simulink model "Modelisation_3_MG_MC_MA_Comparaison_avec_SimMechanics"  (R2016a)
settings: Solver=ode45  StartTime=0.0  StopTime=2.5  RelTol=1e-3
values from neighbouring files (symbols this model uses):
  s = tf('s')    [A_3_LoopShaping.m]    (also in A_4_Hinfini.m = zpk('s'))
  X = [0;0;0;0;0;0;0;0]    [A_1_Data.m]
  Y = [0;0;0;0;0;0;0;0]    [A_1_Data.m]
undefined symbols (not defined in the file or in its folder): sfun3d, Z
libraries: sm_lib x280, nesl_utility x16
(part 7 of 7)

== system Modelisation_3_MG_MC_MA_Comparaison_avec_SimMechanics/SM/Subsystem5/BarreParalleles_3_RIGID/Pi_ce4_Extremetees_1_RIGID ==
  ReferenceFrame : sm_lib/Frames and Transforms/Reference Frame
  Solid : sm_lib/Body Elements/Solid  InertiaType=Custom  Mass=0.0043409919402835973  MassUnits=kg  CenterOfMass=[-6.6394731008193298e-06 -1.3723999560385904 4.9969803448403587]  CenterOfMassUnits=mm  MomentsOfInertia=[0.22208105944838133 0.24049053699814107 0.066049415613599144]  MomentsOfInertiaUnits=kg*mm^2  ProductsOfInertia=[-0.022728057317176146 1.1398156711537084e-07 7.9844492116540505e-07]  ProductsOfInertiaUnits=kg*mm^2  DensityBased=on  Density=1000  DensityUnits=kg/(m^3)  DoExposeReferenceFrame=on  SerializedFrames=<Frames/>  GraphicType=FromGeometry  MarkerShape=Sphere  MarkerSize=10  MarkerSizeUnits=m  GraphicVisPropType=SimpleVisualProperties  GraphicDiffuseColor=[0.59999999999999998 0.59999999999999998 0.59999999999999998]  GraphicSpecularColor=[0.5 0.5 0.5 1.0]  GraphicAmbientColor=[0.15 0.15 0.15 1.0]  GraphicEmissiveColor=[0.0 0.0 0.0 1.0]  GraphicShininess=75  GraphicOpacity=1  GeometryShape=FromFile  RectangleSize=[1 1]  RectangleSizeUnits=m  BrickDimensions=[1 1 1]  BrickDimensionUnits=m  CylinderRadius=1  CylinderRadiusUnits=m  CylinderLength=1  CylinderLengthUnits=m  SphereRadius=1  SphereRadiusUnits=m  EllipsoidRadii=[1 1 1]  EllipsoidRadiiUnits=m  ExtrusionCrossSection=[1 1; -1 1; -1 -1; 1 -1]  ExtrusionCrossSectionUnits=m  ExtrusionLength=1  ExtrusionLengthUnits=m  PolygonNumSides=3  PolygonOuterRadius=1  PolygonOuterRadiusUnits=m  ExtGeomFileType=STL  ExtGeomFileName=Pièce4_Extremetees_Défaut_sldprt.STL  ExtGeomFileUnits=mm  RevolutionCrossSection=[1 1; 1 -1; 2 -1; 2 1]  RevolutionCrossSectionUnits=m  RevolutionExtent=Full  RevolutionAngle=180  RevolutionAngleUnits=deg
  F : PMIOPort  Port=1  Side=Left
  connections:
  F/RConn1 -- ReferenceFrame/RConn1 -- Solid/RConn1

== system Modelisation_3_MG_MC_MA_Comparaison_avec_SimMechanics/SM/Subsystem5/BarreParalleles_3_RIGID/Pi_ce4_Extremetees_2_RIGID ==
  ReferenceFrame : sm_lib/Frames and Transforms/Reference Frame
  Solid : sm_lib/Body Elements/Solid  InertiaType=Custom  Mass=0.0043409919402835973  MassUnits=kg  CenterOfMass=[-6.6394731008193298e-06 -1.3723999560385904 4.9969803448403587]  CenterOfMassUnits=mm  MomentsOfInertia=[0.22208105944838133 0.24049053699814107 0.066049415613599144]  MomentsOfInertiaUnits=kg*mm^2  ProductsOfInertia=[-0.022728057317176146 1.1398156711537084e-07 7.9844492116540505e-07]  ProductsOfInertiaUnits=kg*mm^2  DensityBased=on  Density=1000  DensityUnits=kg/(m^3)  DoExposeReferenceFrame=on  SerializedFrames=<Frames/>  GraphicType=FromGeometry  MarkerShape=Sphere  MarkerSize=10  MarkerSizeUnits=m  GraphicVisPropType=SimpleVisualProperties  GraphicDiffuseColor=[0.59999999999999998 0.59999999999999998 0.59999999999999998]  GraphicSpecularColor=[0.5 0.5 0.5 1.0]  GraphicAmbientColor=[0.15 0.15 0.15 1.0]  GraphicEmissiveColor=[0.0 0.0 0.0 1.0]  GraphicShininess=75  GraphicOpacity=1  GeometryShape=FromFile  RectangleSize=[1 1]  RectangleSizeUnits=m  BrickDimensions=[1 1 1]  BrickDimensionUnits=m  CylinderRadius=1  CylinderRadiusUnits=m  CylinderLength=1  CylinderLengthUnits=m  SphereRadius=1  SphereRadiusUnits=m  EllipsoidRadii=[1 1 1]  EllipsoidRadiiUnits=m  ExtrusionCrossSection=[1 1; -1 1; -1 -1; 1 -1]  ExtrusionCrossSectionUnits=m  ExtrusionLength=1  ExtrusionLengthUnits=m  PolygonNumSides=3  PolygonOuterRadius=1  PolygonOuterRadiusUnits=m  ExtGeomFileType=STL  ExtGeomFileName=Pièce4_Extremetees_Défaut_sldprt.STL  ExtGeomFileUnits=mm  RevolutionCrossSection=[1 1; 1 -1; 2 -1; 2 1]  RevolutionCrossSectionUnits=m  RevolutionExtent=Full  RevolutionAngle=180  RevolutionAngleUnits=deg
  F : PMIOPort  Port=1  Side=Left
  connections:
  F/RConn1 -- ReferenceFrame/RConn1 -- Solid/RConn1

== system Modelisation_3_MG_MC_MA_Comparaison_avec_SimMechanics/SM/Subsystem5/BarreParalleles_3_RIGID/Pi_ce4_Tube_1_RIGID ==
  ReferenceFrame : sm_lib/Frames and Transforms/Reference Frame
  Solid : sm_lib/Body Elements/Solid  InertiaType=Custom  Mass=0.0056953775725032503  MassUnits=kg  CenterOfMass=[-4.1460122344799134e-11 2.6332345173922464e-08 157.00037492761294]  CenterOfMassUnits=mm  MomentsOfInertia=[46.656669534748204 46.656784060773653 0.060513437161415488]  MomentsOfInertiaUnits=kg*mm^2  ProductsOfInertia=[4.4271388779002391e-06 -1.0344554341986986e-06 -6.5578304138838094e-07]  ProductsOfInertiaUnits=kg*mm^2  DensityBased=on  Density=1000  DensityUnits=kg/(m^3)  DoExposeReferenceFrame=on  SerializedFrames=<Frames/>  GraphicType=FromGeometry  MarkerShape=Sphere  MarkerSize=10  MarkerSizeUnits=m  GraphicVisPropType=SimpleVisualProperties  GraphicDiffuseColor=[1 1 1]  GraphicSpecularColor=[0.5 0.5 0.5 1.0]  GraphicAmbientColor=[0.15 0.15 0.15 1.0]  GraphicEmissiveColor=[0.0 0.0 0.0 1.0]  GraphicShininess=75  GraphicOpacity=1  GeometryShape=FromFile  RectangleSize=[1 1]  RectangleSizeUnits=m  BrickDimensions=[1 1 1]  BrickDimensionUnits=m  CylinderRadius=1  CylinderRadiusUnits=m  CylinderLength=1  CylinderLengthUnits=m  SphereRadius=1  SphereRadiusUnits=m  EllipsoidRadii=[1 1 1]  EllipsoidRadiiUnits=m  ExtrusionCrossSection=[1 1; -1 1; -1 -1; 1 -1]  ExtrusionCrossSectionUnits=m  ExtrusionLength=1  ExtrusionLengthUnits=m  PolygonNumSides=3  PolygonOuterRadius=1  PolygonOuterRadiusUnits=m  ExtGeomFileType=STL  ExtGeomFileName=Pièce4_Tube_Défaut_sldprt.STL  ExtGeomFileUnits=mm  RevolutionCrossSection=[1 1; 1 -1; 2 -1; 2 1]  RevolutionCrossSectionUnits=m  RevolutionExtent=Full  RevolutionAngle=180  RevolutionAngleUnits=deg
  F : PMIOPort  Port=1  Side=Left
  connections:
  F/RConn1 -- ReferenceFrame/RConn1 -- Solid/RConn1

== system Modelisation_3_MG_MC_MA_Comparaison_avec_SimMechanics/SM/Subsystem5/BarreParalleles_4_RIGID/Pi_ce4_Extremetees_1_RIGID ==
  ReferenceFrame : sm_lib/Frames and Transforms/Reference Frame
  Solid : sm_lib/Body Elements/Solid  InertiaType=Custom  Mass=0.0043409919402835973  MassUnits=kg  CenterOfMass=[-6.6394731008193298e-06 -1.3723999560385904 4.9969803448403587]  CenterOfMassUnits=mm  MomentsOfInertia=[0.22208105944838133 0.24049053699814107 0.066049415613599144]  MomentsOfInertiaUnits=kg*mm^2  ProductsOfInertia=[-0.022728057317176146 1.1398156711537084e-07 7.9844492116540505e-07]  ProductsOfInertiaUnits=kg*mm^2  DensityBased=on  Density=1000  DensityUnits=kg/(m^3)  DoExposeReferenceFrame=on  SerializedFrames=<Frames/>  GraphicType=FromGeometry  MarkerShape=Sphere  MarkerSize=10  MarkerSizeUnits=m  GraphicVisPropType=SimpleVisualProperties  GraphicDiffuseColor=[0.59999999999999998 0.59999999999999998 0.59999999999999998]  GraphicSpecularColor=[0.5 0.5 0.5 1.0]  GraphicAmbientColor=[0.15 0.15 0.15 1.0]  GraphicEmissiveColor=[0.0 0.0 0.0 1.0]  GraphicShininess=75  GraphicOpacity=1  GeometryShape=FromFile  RectangleSize=[1 1]  RectangleSizeUnits=m  BrickDimensions=[1 1 1]  BrickDimensionUnits=m  CylinderRadius=1  CylinderRadiusUnits=m  CylinderLength=1  CylinderLengthUnits=m  SphereRadius=1  SphereRadiusUnits=m  EllipsoidRadii=[1 1 1]  EllipsoidRadiiUnits=m  ExtrusionCrossSection=[1 1; -1 1; -1 -1; 1 -1]  ExtrusionCrossSectionUnits=m  ExtrusionLength=1  ExtrusionLengthUnits=m  PolygonNumSides=3  PolygonOuterRadius=1  PolygonOuterRadiusUnits=m  ExtGeomFileType=STL  ExtGeomFileName=Pièce4_Extremetees_Défaut_sldprt.STL  ExtGeomFileUnits=mm  RevolutionCrossSection=[1 1; 1 -1; 2 -1; 2 1]  RevolutionCrossSectionUnits=m  RevolutionExtent=Full  RevolutionAngle=180  RevolutionAngleUnits=deg
  F : PMIOPort  Port=1  Side=Left
  connections:
  F/RConn1 -- ReferenceFrame/RConn1 -- Solid/RConn1

== system Modelisation_3_MG_MC_MA_Comparaison_avec_SimMechanics/SM/Subsystem5/BarreParalleles_4_RIGID/Pi_ce4_Extremetees_2_RIGID ==
  ReferenceFrame : sm_lib/Frames and Transforms/Reference Frame
  Solid : sm_lib/Body Elements/Solid  InertiaType=Custom  Mass=0.0043409919402835973  MassUnits=kg  CenterOfMass=[-6.6394731008193298e-06 -1.3723999560385904 4.9969803448403587]  CenterOfMassUnits=mm  MomentsOfInertia=[0.22208105944838133 0.24049053699814107 0.066049415613599144]  MomentsOfInertiaUnits=kg*mm^2  ProductsOfInertia=[-0.022728057317176146 1.1398156711537084e-07 7.9844492116540505e-07]  ProductsOfInertiaUnits=kg*mm^2  DensityBased=on  Density=1000  DensityUnits=kg/(m^3)  DoExposeReferenceFrame=on  SerializedFrames=<Frames/>  GraphicType=FromGeometry  MarkerShape=Sphere  MarkerSize=10  MarkerSizeUnits=m  GraphicVisPropType=SimpleVisualProperties  GraphicDiffuseColor=[0.59999999999999998 0.59999999999999998 0.59999999999999998]  GraphicSpecularColor=[0.5 0.5 0.5 1.0]  GraphicAmbientColor=[0.15 0.15 0.15 1.0]  GraphicEmissiveColor=[0.0 0.0 0.0 1.0]  GraphicShininess=75  GraphicOpacity=1  GeometryShape=FromFile  RectangleSize=[1 1]  RectangleSizeUnits=m  BrickDimensions=[1 1 1]  BrickDimensionUnits=m  CylinderRadius=1  CylinderRadiusUnits=m  CylinderLength=1  CylinderLengthUnits=m  SphereRadius=1  SphereRadiusUnits=m  EllipsoidRadii=[1 1 1]  EllipsoidRadiiUnits=m  ExtrusionCrossSection=[1 1; -1 1; -1 -1; 1 -1]  ExtrusionCrossSectionUnits=m  ExtrusionLength=1  ExtrusionLengthUnits=m  PolygonNumSides=3  PolygonOuterRadius=1  PolygonOuterRadiusUnits=m  ExtGeomFileType=STL  ExtGeomFileName=Pièce4_Extremetees_Défaut_sldprt.STL  ExtGeomFileUnits=mm  RevolutionCrossSection=[1 1; 1 -1; 2 -1; 2 1]  RevolutionCrossSectionUnits=m  RevolutionExtent=Full  RevolutionAngle=180  RevolutionAngleUnits=deg
  F : PMIOPort  Port=1  Side=Left
  connections:
  F/RConn1 -- ReferenceFrame/RConn1 -- Solid/RConn1

== system Modelisation_3_MG_MC_MA_Comparaison_avec_SimMechanics/SM/Subsystem5/BarreParalleles_4_RIGID/Pi_ce4_Tube_1_RIGID ==
  ReferenceFrame : sm_lib/Frames and Transforms/Reference Frame
  Solid : sm_lib/Body Elements/Solid  InertiaType=Custom  Mass=0.0056953775725032503  MassUnits=kg  CenterOfMass=[-4.1460122344799134e-11 2.6332345173922464e-08 157.00037492761294]  CenterOfMassUnits=mm  MomentsOfInertia=[46.656669534748204 46.656784060773653 0.060513437161415488]  MomentsOfInertiaUnits=kg*mm^2  ProductsOfInertia=[4.4271388779002391e-06 -1.0344554341986986e-06 -6.5578304138838094e-07]  ProductsOfInertiaUnits=kg*mm^2  DensityBased=on  Density=1000  DensityUnits=kg/(m^3)  DoExposeReferenceFrame=on  SerializedFrames=<Frames/>  GraphicType=FromGeometry  MarkerShape=Sphere  MarkerSize=10  MarkerSizeUnits=m  GraphicVisPropType=SimpleVisualProperties  GraphicDiffuseColor=[1 1 1]  GraphicSpecularColor=[0.5 0.5 0.5 1.0]  GraphicAmbientColor=[0.15 0.15 0.15 1.0]  GraphicEmissiveColor=[0.0 0.0 0.0 1.0]  GraphicShininess=75  GraphicOpacity=1  GeometryShape=FromFile  RectangleSize=[1 1]  RectangleSizeUnits=m  BrickDimensions=[1 1 1]  BrickDimensionUnits=m  CylinderRadius=1  CylinderRadiusUnits=m  CylinderLength=1  CylinderLengthUnits=m  SphereRadius=1  SphereRadiusUnits=m  EllipsoidRadii=[1 1 1]  EllipsoidRadiiUnits=m  ExtrusionCrossSection=[1 1; -1 1; -1 -1; 1 -1]  ExtrusionCrossSectionUnits=m  ExtrusionLength=1  ExtrusionLengthUnits=m  PolygonNumSides=3  PolygonOuterRadius=1  PolygonOuterRadiusUnits=m  ExtGeomFileType=STL  ExtGeomFileName=Pièce4_Tube_Défaut_sldprt.STL  ExtGeomFileUnits=mm  RevolutionCrossSection=[1 1; 1 -1; 2 -1; 2 1]  RevolutionCrossSectionUnits=m  RevolutionExtent=Full  RevolutionAngle=180  RevolutionAngleUnits=deg
  F : PMIOPort  Port=1  Side=Left
  connections:
  F/RConn1 -- ReferenceFrame/RConn1 -- Solid/RConn1

== matlab function Modelisation_3_MG_MC_MA_Comparaison_avec_SimMechanics/SM/MCI ==
  data: alpha input; dalpha input; d2alpha input; alpha_ output; dalpha_ output; d2alpha_ output
    function [alpha_, dalpha_,d2alpha_]= fcn(alpha, dalpha,d2alpha)

   alpha_= -alpha + [0.0651 ; 0.0651 ;0.0651 ] ;  %alpha_= -alpha ;
   dalpha_= -dalpha;
   d2alpha_= -d2alpha ;

== matlab function Modelisation_3_MG_MC_MA_Comparaison_avec_SimMechanics/Modele inverse ==
  data: P input; dP input; d2P input; alpha output; dalpha output; d2alpha output
    function [alpha, dalpha,d2alpha]= fcn(P,dP,d2P)

    l1 = 0.19992; 
    l2 = 0.334; 
    r = 0.126; 
    phi2 = 2*pi/3;
    phi3 = 4*pi/3;

    %% Expression de P dans Ri
    % l'expression P1 dP1 et d2P1 ne se changent pas
    A2=[cos(phi2) sin(phi2) 0
        -sin(phi2) cos(phi2) 0
        0            0      1 ]; 
    A3=[cos(phi3) sin(phi3) 0
        -sin(phi3) cos(phi3) 0
        0            0      1 ];
     P2=A2*P; dP2=A2*dP; d2P2=A2*d2P; 
     P3=A3*P ; dP3=A3*dP ; d2P3=A3*d2P ; 
        
    x1=P(1); y1=P(2) ; z1=P(3) ; 
    x2=P2(1); y2=P2(2) ; z2=P2(3) ;
    x3=P3(1); y3=P3(2) ; z3=P3(3) ;
    % Notation de dP :
    dx1=dP(1); dy1=dP(2) ; dz1=dP(3) ; 
    dx2=dP2(1); dy2=dP2(2) ; dz2=dP2(3) ; 
    dx3=dP3(1); dy3=dP3(2) ; dz3=dP3(3) ; 
    % Notation de d2P :
    d2x1=d2P(1); d2y1=d2P(2) ; d2z1=d2P(3) ;
    d2x2=d2P2(1); d2y2=d2P2(2) ; d2z2=d2P2(3) ;
    d2x3=d2P3(1); d2y3=d2P3(2) ; d2z3=d2P3(3) ;
         

    %% Parametres du Triangle AiCiBi :
    % Triangle 1 :
    AB1=sqrt(z1^2+(x1-r)^2);
    e1=sqrt(l2^2-y1^2); 
    AB2=sqrt(z2^2+(x2-r)^2);
    e2=sqrt(l2^2-y2^2);
    AB3=sqrt(z3^2+(x3-r)^2);
    e3=sqrt(l2^2-y3^2);

    %% calcul de alpha1
    beta1=atan2(-z1,x1-r);
    delta1=acos((AB1^2 + l1^2 - e1^2)/(2*l1*AB1));
    alpha1=beta1-delta1; 


    %% calcul de alpha2
    beta2=atan2(-z2,x2-r);
    delta2=acos((AB2^2 + l1^2 - e2^2)/(2*l1*AB2));
    alpha2=beta2-delta2; 


    %% calcul de alpha3
    beta3=atan2(-z3,x3-r);
    delta3=acos((AB3^2 + l1^2 - e3^2)/(2*l1*AB3));
    alpha3=beta3-delta3; 

% Tranformation au Deg
alpha=[alpha1;alpha2;alpha3]; % first solution


%% =================== Calcule de dalpha_i ====================================

% ---------------------------- Calcul de dAlpha1 ----------------------
% Calcule de dDelta1 :
BH1 = AB1-l1*cos(delta1);
D1=l1*AB1*sin(delta1) ;
dDelta1X = -BH1*(x1-r)/AB1/D1 ; 
dDelta1Y = -y1/D1 ; 
dDelta1Z = -BH1*z1/AB1/D1 ; 
Gdelta1=  [ dDelta1X , dDelta1Y , dDelta1Z] ;
dDelta1 = Gdelta1*dP ;
% Calcule de dBeta1 :
dBeta1Z=-(x1-r)/AB1^2 ; dBeta1X=z1/AB1^2 ;
Gbeta1=[ dBeta1X ,  0 , dBeta1Z] ;
dBeta1 = Gbeta1*dP;
% Calcule de dAlpha1 :
Galpha1=Gbeta1-Gdelta1 ;
dAlpha1 = Galpha1*dP ;

% ---------------------------- Calcul de dAlpha2 ----------------------
% Calcule de dDelta2 :
BH2 = AB2-l1*cos(delta2);
D2=l1*AB2*sin(delta2) ;
dDelta2X = -BH2*(x2-r)/AB2/D2 ; 
dDelta2Y = -y2/D2 ; 
dDelta2Z = -BH2*z2/AB2/D2 ; 
Gdelta2=  [ dDelta2X , dDelta2Y , dDelta2Z] ;
dDelta2 = Gdelta2*dP2 ;
% Calcule de dBeta2 :
dBeta2Z=-(x2-r)/AB2^2 ; dBeta2X=z2/AB2^2 ;
Gbeta2=[ dBeta2X ,  0 , dBeta2Z] ;
dBeta2 = Gbeta2*dP2;
% Calcule de dAlpha2 :
Galpha2=Gbeta2-Gdelta2 ;
dAlpha2 = Galpha2*dP2 ;

% ---------------------------- Calcul de dAlpha3 ----------------------
% Calcule de dDelta2 :
BH3 = AB3-l1*cos(delta3);
D3=l1*AB3*sin(delta3) ;
dDelta3X = -BH3*(x3-r)/AB3/D3 ; 
dDelta3Y = -y3/D3 ; 
dDelta3Z = -BH3*z3/AB3/D3 ; 
Gdelta3=  [ dDelta3X , dDelta3Y , dDelta3Z] ;
dDelta3 = Gdelta3*dP3 ;
% Calcule de dBeta3:
dBeta3Z=-(x3-r)/AB3^2 ; dBeta2X=z3/AB3^2 ;
Gbeta3=[ dBeta2X ,  0 , dBeta3Z] ;
dBeta3 = Gbeta3*dP3;
% Calcule de dAlpha3 :
Galpha3=Gbeta3-Gdelta3 ;
dAlpha3 = Galpha3*dP3 ;

dalpha=[ dAlpha1 ; dAlpha2 ; dAlpha3 ];

%% ===================== Calcule de d2alpha_i =================================
 
% ---------------------------- Calcul de d2Alpha1 ----------------------
% Calcule de d2Gama1 :
CH1=l1*sin(delta1);
AH1=l1*cos(delta1) ;
d2Delta1XX = -BH1*(x1-r)^2/(AB1^3*D1)*( AH1*e1^2/(BH1*CH1^2) + (AB1/(x1-r))^2 - 2 ) ;
d2Delta1YY = - (1+y1^2*AH1*AB1/D1^2 )  /D1;
d2Delta1ZZ  = -BH1*z1^2/(AB1^3*D1)*( AH1*e1^2/(BH1*CH1^2) + (AB1/z1)^2 -2 ) ;
d2Delta1XY = y1*(x1-r)*(CH1^2-AH1*BH1)/D1^3 ;
d2Delta1XZ = -BH1*(x1-r)*z1/(AB1^3*D1)*( AH1*e1^2/(BH1*CH1^2) - 2 ) ;
d2Delta1YZ = y1*z1*(CH1^2-AH1*BH1)/D1^3 ; 
Hdelta1=[ d2Delta1XX,d2Delta1XY,d2Delta1XZ ; d2Delta1XY, d2Delta1YY,d2Delta1YZ ;d2Delta1XZ , d2Delta1YZ,d2Delta1ZZ] ;
d2Delta1=dP'*Hdelta1*dP +  Gdelta1*d2P ; 
%Calcule de dBeta 1:
d2Beta1XX=-2*(x1-r)*z1/AB1^4 ; d2Beta1ZZ=-d2Beta1XX ; d2Beta1XZ = ((x1-r)^2-z1^2)/AB1^4 ;
Hbeta1= [d2Beta1XX , 0, d2Beta1XZ ; 0, 0, 0 ; d2Beta1XZ , 0 , d2Beta1ZZ ] ;
d2Beta1=dP'*Hbeta1*dP + Gbeta1*d2P;
%Calcule de dAlpha1 :
Halpha1= Hbeta1 - Hdelta1; 
d2Alpha1=dP'*Halpha1*dP + Galpha1*d2P;

% ---------------------------- Calcul de d2Alpha2 ----------------------
% Calcule de d2Gama1 :
CH2=l1*sin(delta2);
AH2=l1*cos(delta2) ;
d2Delta2XX = -BH2*(x2-r)^2/(AB2^3*D2)*( AH2*e2^2/(BH2*CH2^2) + (AB2/(x2-r))^2 - 2 ) ;
d2Delta2YY = - (1+y2^2*AH2*AB2/D2^2 )  /D2;
d2Delta2ZZ  = -BH2*z2^2/(AB2^3*D2)*( AH2*e2^2/(BH2*CH2^2) + (AB2/z2)^2 -2 ) ;
d2Delta2XY = y2*(x2-r)*(CH2^2-AH2*BH2)/D2^3 ;
d2Delta2XZ = -BH2*(x2-r)*z2/(AB2^3*D2)*( AH2*e2^2/(BH2*CH2^2) - 2 ) ;
d2Delta2YZ = y2*z2*(CH2^2-AH2*BH2)/D2^3 ; 
Hdelta2=[ d2Delta2XX,d2Delta2XY,d2Delta2XZ ; d2Delta2XY, d2Delta2YY,d2Delta2YZ ;d2Delta2XZ , d2Delta2YZ,d2Delta2ZZ] ;
d2Delta1=dP2'*Hdelta2*dP2 +  Gdelta2*d2P2 ; 
%Calcule de dBeta2:
d2Beta2XX=-2*(x2-r)*z2/AB2^4 ; d2Beta2ZZ=-d2Beta2XX ; d2Beta2XZ = ((x2-r)^2-z2^2)/AB2^4 ;
Hbeta2= [d2Beta2XX , 0, d2Beta2XZ ; 0, 0, 0 ; d2Beta2XZ , 0 , d2Beta2ZZ ] ;
d2Beta2=dP2'*Hbeta2*dP2 + Gbeta2*d2P2;
%Calcule de dAlpha2 :
Halpha2= Hbeta2 - Hdelta2; 
d2Alpha2=dP2'*Halpha2*dP2 + Galpha2*d2P2;

% ---------------------------- Calcul de d2Alpha3 ----------------------
% Calcule de d2Gama3 :
CH3=l1*sin(delta3);
AH3=l1*cos(delta3) ;
d2Delta3XX = -BH3*(x3-r)^2/(AB3^3*D3)*( AH3*e3^2/(BH3*CH3^2) + (AB3/(x3-r))^2 - 2 ) ;
d2Delta3YY = - (1+y3^2*AH3*AB3/D3^2 )  /D3;
d2Delta3ZZ  = -BH3*z3^2/(AB3^3*D3)*( AH3*e3^2/(BH3*CH3^2) + (AB3/z3)^2 -2 ) ;
d2Delta3XY = y3*(x3-r)*(CH3^2-AH3*BH3)/D3^3 ;
d2Delta3XZ = -BH3*(x3-r)*z3/(AB3^3*D3)*( AH3*e3^2/(BH3*CH3^2) - 2 ) ;
d2Delta3YZ = y3*z3*(CH3^2-AH3*BH3)/D3^3 ; 
Hdelta3=[ d2Delta3XX,d2Delta3XY,d2Delta3XZ ; d2Delta3XY, d2Delta3YY,d2Delta3YZ ;d2Delta3XZ , d2Delta3YZ,d2Delta3ZZ] ;
d2Delta3=dP3'*Hdelta3*dP3 +  Gdelta3*d2P3 ; 
%Calcule de dBeta3:
d2Beta3XX=-2*(x3-r)*z3/AB3^4 ; d2Beta3ZZ=-d2Beta3XX ; d2Beta3XZ = ((x3-r)^2-z3^2)/AB3^4 ;
Hbeta3= [d2Beta3XX , 0, d2Beta3XZ ; 0, 0, 0 ; d2Beta3XZ , 0 , d2Beta3ZZ ] ;
d2Beta2=dP3'*Hbeta3*dP3 + Gbeta3*d2P3;
%Calcule de dAlpha3 :
Halpha3= Hbeta3 - Hdelta3; 
d2Alpha3=dP3'*Halpha3*dP3 + Galpha3*d2P3;

d2alpha=[d2Alpha1 ; d2Alpha2 ; d2Alpha3];

%%  Autres formule pour calculer d2Delta :
% % ---------------------------- Calcul de d2Alpha1 ----------------------
% % Calcule de d2Delta1 :
% dAB1 = ( z1*dz1 + (x1-r)*dx1 )/AB1 ;
% d2AB1 = (dz1^2 + z1*d2z1 + dx1^2 + (x1-r)*d2x1 -dAB1^2 )/AB1 ;
% de1=(-y1*dy1)/e1 ;
% d2e1 = -(dy1^2 + y1*d2y1 + de1^2)/e1 ;
% d2Delta1=( dAB1^2 + AB1*d2AB1 - de1^2 - e1*d2e1 -l1*(d2AB1*cos(delta1)-2*dAB1*sin(delta1)*dDelta1 - AB1*cos(delta1)*dDelta1^2) )  /(-l1*AB1*sin(delta1));

== matlab function Modelisation_3_MG_MC_MA_Comparaison_avec_SimMechanics/Modele Directe ==
  data: P output; alpha input; dalpha input; dP output; d2P output; d2alpha input
function [P,dP,d2P]= fcn(alpha,dalpha,d2alpha)

% alpha=alpha*pi/180;
% dalpha=dalpha*pi/180;
% d2alpha=d2alpha*pi/180;
alpha1=alpha(1) ;alpha2=alpha(2) ; alpha3=alpha(3) ;
dalpha1=dalpha(1) ;dalpha2=dalpha(2) ; dalpha3=dalpha(3) ;
d2alpha1=d2alpha(1) ;d2alpha2=d2alpha(2) ; d2alpha3=d2alpha(3) ;
%% Remarque: une letrre majiscule signifie un point ou un vecteur 
% tandit que un miniscule signifie la norme
%% les constantes
l1 = 0.19992; 
l2 = 0.334; 
r = 0.126; 
phi2 = 2*pi/3;
phi3 = 4*pi/3;
% Fin
%% les points Ci :
OC1=[r+l1*cos(alpha1) ; 0 ; -l1*sin(alpha1) ]; 
OC2=[(r+l1*cos(alpha2))*cos(phi2) ; (r+l1*cos(alpha2))*sin(phi2) ; -l1*sin(alpha2) ]; 
OC3=[(r+l1*cos(alpha3))*cos(phi3) ; (r+l1*cos(alpha3))*sin(phi3) ; -l1*sin(alpha3) ]; 
%% Les veccteurs CiCj :
C1C2=OC2-OC1; C2C3=OC3-OC2 ; C3C1=OC1-OC3;
%% vitesses de point Ci et CiCj:
% dC1= Q1*dAlpha1;
Q1=[-l1*sin(alpha1) ; 0 ; -l1*cos(alpha1)] ; 
Q2=[-l1*sin(alpha2)*cos(phi2) ; -l1*sin(alpha2)*sin(phi2) ; -l1*cos(alpha2)] ;
Q3=[-l1*sin(alpha3)*cos(phi3) ; -l1*sin(alpha3)*sin(phi3) ; -l1*cos(alpha3)] ;
dOC1=Q1*dalpha1 ;
dOC2=Q2*dalpha2 ;
dOC3=Q3*dalpha3 ;
dC1C2=dOC2-dOC1 ; dC2C3=dOC3-dOC2 ; dC3C1=dOC1-dOC3 ;

%% Les longueurs a,b,et c:
a=sqrt(C1C2'*C1C2);
b=sqrt(C2C3'*C2C3);
c=sqrt(C3C1'*C3C1);

%% Calcule de R et s :
p=a+b+c ; % le perimetre
p1=p-2*a ; p2=p-2*b ;  p3=p-2*c ; 
R=a*b*c/sqrt(p*p1*p2*p3); % le Rayon du C1C2C3
s=a*b*c/(2*R); % La surface
V1=C1C2/a; % les vecteures unitaires portes sur les segments
V2=C2C3/b;
V3=C3C1/c;
%% Calcule de n et w:
n=cross(C3C1,C1C2)/s ; % le Vecteur normale
w = cross(n,V1) ;
%% les segments  tl=|TK| , ml=|ML| ,lp=|LP|
tl=sqrt(R^2-(a/2)^2);
% ml=sqrt(R^2-(b/2)^2);
% kl=sqrt(R^2-(c/2)^2);
lp=sqrt(l2^2-R^2) ;
%% les vitess de a,b,et c:
da=V1'*dC1C2;
db=V2'*dC2C3;
dc=V3'*dC3C1;
%% Calcule de dR:
dp=da+db+dc ;
dp1=dp-2*da ; dp2=dp-2*db ; dp3=dp-2*dc ;
dR = ( da/a + db/b + dc/c - 0.5*( dp/p + dp1/p1 + dp2/p2 + dp3/p3 ))*R ;
%dR = ( 1 - 4*R*tl/b/c)*R*da/a + (1-4*R*ml/a/c)*R*db/b + (1-4*R*kl/a/b)*R*dc/c ;
%% Calcule de :
dtl=(R*dR-a*da/4)/tl ;
dlp  = -R*dR/lp ;
ds = (da/a + db/b + dc/c - dR/R)*s ;
dV1=(dC1C2-da*V1)/a ;

dS = cross(dC3C1,C1C2) + cross(C3C1,dC1C2) ;
dn= (dS-ds*n)/s ;
dw=sign(-a*a+c*c+b*b)*(cross(dn,V1) + cross(n,dV1)) ;
% Calcule de P :
OL = (OC1+OC2)/2 + tl*w;
P = OL-lp*n ;
% Calcule de dP :
dOT = (dOC2 + dOC1)/2 ; 
dTL = dtl*w + tl*dw ;
dLP = -dlp*n - lp*dn ; 
dP = dOT + dTL + dLP ; 

%==================== d2OP en fonction de  d2alpha =======================
  %% L'acceleration de OCi  CiCj:
dQ1=[-l1*cos(alpha1) ; 0 ; l1*sin(alpha1)] ; dQ1t= dQ1*dalpha1 ;
dQ2=[-l1*cos(alpha2)*cos(phi2) ; -l1*cos(alpha2)*sin(phi2) ; l1*sin(alpha2)] ;dQ2t= dQ2*dalpha2 ;
dQ3=[-l1*cos(alpha3)*cos(phi3) ; -l1*cos(alpha3)*sin(phi3) ; l1*sin(alpha3)] ;dQ3t= dQ3*dalpha3 ;

d2C1 = dQ1*dalpha1^2 + Q1*d2alpha1;
d2C2 = dQ2*dalpha2^2 + Q2*d2alpha2;
d2C3 = dQ3*dalpha3^2 + Q3*d2alpha3;
d2C1C2=d2C2-d2C1 ;
d2C2C3=d2C3-d2C2 ; d2C3C1=d2C1-d2C3 ;
%% Les accelerations de a,b et c :
d2a = (d2C1C2'*C1C2 + dC1C2'*dC1C2 - da^2)/a ;
d2b = (d2C2C3'*C2C3 + dC2C3'*dC2C3 - db^2)/b ;
d2c = (d2C3C1'*C3C1 + dC3C1'*dC3C1 - dc^2)/c ;
%% L'acceleration de V1 :
d2V1=(d2C1C2 - 2*da*dV1 - d2a*V1)/a ;
%% L'acceleration de R :
d2p=d2a+d2b+d2c;
d2p1=d2p-2*d2a ; d2p2=d2p-2*d2b ; d2p3=d2p-2*d2c ;
d2R = ( d2a/a + d2b/b + d2c/c - 0.5*(d2p/p +  d2p1/p1 +  d2p2/p2 +  d2p3/p3 ) - (da/a)^2 -(db/b)^2 -(dc/c)^2 +0.5*( (dp/p)^2 +(dp1/p1)^2 +(dp2/p2)^2 +(dp3/p3)^2 ) +(dR/R)^2 )*R;
%% L'acceleration de S et s :
d2s = (d2a/a + d2b/b + d2c/c -d2R/R - (da/a)^2 -(db/b)^2 -(dc/c)^2 +(dR/R)^2 + (ds/s)^2)*s ;
d2S=cross(d2C3C1,C1C2) + 2*cross(dC3C1,dC1C2) + cross(C3C1,d2C1C2) ;
%% L'acceleraion de n et w ;
d2n=(d2S - d2s*n - 2*ds*dn)/s ;
d2w= sign(-a*a+c*c+b*b)*(cross(d2n,V1) +2*cross(dn,dV1) + cross(n,d2V1)) ;

%% Calcule de d2OT :
d2OT = (d2C1+d2C2)/2 ;
%% Calcule de d2TL ;
d2tl = (d2R*R + dR^2 - ( d2a*a + da^2 )/4 - dtl^2 )/tl ;
d2TL =d2tl*w + 2*dtl*dw + tl*d2w ;
%% Calcule de d2LP :
d2lp = -(d2R*R + dR^2 + dlp^2)/lp ;
d2LP = -d2lp*n -2*dlp*dn - lp*d2n ;
 
%% Calcule de d2P :
d2P = d2OT + d2TL + d2LP ;
% les commemtaires v=|V|

== matlab function Modelisation_3_MG_MC_MA_Comparaison_avec_SimMechanics/Trajectoir1 ==
  data: ne input; P output; dP output; d2P output; t input
function [P,dP,d2P]= fcn(ne,t)

%% Menu
% 1 ==> Ligne horizontal
% 2==>  Ligne suivant l'axe oz
% 3==> Cercle
% 4==> Ligne x=y
 z0=-0.08789  ; zpi=-0.3;
B= (z0+zpi)/2 ; A= (z0-zpi)/2 ; 
f = 9; f2 = 5 ;
R=0.3;
%% vers le Plan Z=-0.3
if (t<pi/f && (ne == 1 || ne == 3 ||  ne == 0 || ne == 4 || ne == 5 ||  ne == 6))
n= 2 ; 
elseif( (ne == 4 || ne == 5 ||  ne == 6)  &&  (t<3*pi/2/f) ) % vers le point (0 , R , -0.3)
n=1 ;
else
n =ne ;
end

%% le trajecoir
switch n
    
    case 0
        
        % La position
        x = R*sin(f*t)  ; y=0 ;
        z=  zpi ;
        P = [ x ; y ; z ];
        % La vitess
        dx = f*R*cos(f*t)  ; dy=0 ;
        dz= 0 ;
        dP = [ dx ; dy ; dz ];
        % L'acceleration :
        d2x = -f^2*R*sin(f*t) ; d2y=0 ;
        d2z =  0;
        d2P = [ d2x ; d2y ; d2z ];
        % L'a _coup :
        d3x = -f^3*R*cos(f*t) ; d3y=0 ;
        d3z =  0;
        d3P = [ d3x ; d3y ; d3z ];
    case 1   
        % La position
        y = R*sin(f*t)  ; x=0 ;
        z= zpi  ;
        P = [ x ; y ; z ];
        % La vitess
        dy = f*R*cos(f*t)  ; dx=0 ;
        dz= 0 ;
        dP = [ dx ; dy ; dz ];
        % L'acceleration :
        d2y = -f^2*R*sin(f*t) ; d2x=0 ;
        d2z =  0;
        d2P = [ d2x ; d2y ; d2z ];
        % L'a _coup :
        d3y = -f^3*R*cos(f*t) ; d3x=0 ;
        d3z =  0;
        d3P = [ d3x ; d3y ; d3z ];
    case 2
        % La position 
        x = 0 ; y=0 ;
        z= A*cos(f*t) + B ; 
        P = [ x ; y ; z ];
        % La vitess
        dx = 0 ; dy=0 ;
        dz= -f*A*sin(f*t) ;
        dP = [ dx ; dy ; dz ];
        % L'acceleration :
        d2x = 0 ; d2y=0 ;
        d2z = -f^2*A*cos(f*t) ;
        d2P = [ d2x ; d2y ; d2z ];
        % L a_coup (jerk) :
        d3x = 0 ; d3y=0 ;
        d3z = f^3*A*sin(f*t) ;
        d3P = [ d3x ; d3y ; d3z ];
        
        %%
    case 3
        R=0.12;
        y = R*sin(f*t)  ; x=2*y;
        z= zpi  ;
        P = [ x ; y ; z ];
        % La vitess
        dy = f*R*cos(f*t)  ; dx=2*dy ;
        dz= 0 ;
        dP = [ dx ; dy ; dz ];
        % L'acceleration :
        d2y = -f^2*R*sin(f*t) ; d2x=2*d2y ;
        d2z =  0;
        d2P = [ d2x ; d2y ; d2z ];
        % L'a _coup :
        d3y = -f^3*R*cos(f*t) ; d3x=2*d3y ;
        d3z =  0;
        d3P = [ d3x ; d3y ; d3z ];
    case 4 % Cerecl XY
        x=R*cos(f*t) ; y=R*sin(f*t) ; z=zpi  ;
        dx=-f*R*sin(f*t) ; dy=f*R*cos(f*t)  ;  dz=0;
        d2x=-f^2*R*cos(f*t) ; d2y=-f^2*R*sin(f*t)  ;  d2z=0;
        P=[x ; y ; z];
        dP=[dx ; dy ; dz];
        d2P=[d2x ; d2y ; d2z];
        % L'a _coup :
        d3x=f^3*R*sin(f*t) ; d3y=-f^3*R*cos(f*t)  ;  d3z=0;
        d3P=[d3x ; d3y ; d3z];
        
    case 5 % ZY   
        x=0 ; y=R*sin(f*t) ; z=0.5*R*cos(f*t) + zpi  ;
        dx=0 ; dy=f*R*cos(f*t)  ;  dz=-f*R*sin(f*t);
        d2x=0 ; d2y=-f^2*R*sin(f*t)  ;  d2z=-f^2*R*cos(f*t);
        P=[x ; y ; z];
        dP=[dx ; dy ; dz];
        d2P=[d2x ; d2y ; d2z];
        d3x=0 ; d3y=-f^3*R*cos(f*t)  ;  d3z=f^3*R*sin(f*t);
        d3P=[d3x ; d3y ; d3z];
%     case 6 %Cercle ZX
%         y=0 ; x=R*sin(f*t) ; z=R*cos(f*t) +zpi;
%         dy=0 ; dx=f*R*cos(f*t)  ;  dz=-f*R*sin(f*t);
%         d2y=0 ; d2x=-f^2*R*sin(f*t)  ;  d2z=-f^2*R*cos(f*t);
%         d3y=0 ; d3x=-f^3*R*cos(f*t)  ;  d3z=f^3*R*sin(f*t);
%         P=[x ; y ; z];
%         dP=[dx ; dy ; dz];
%         d2P=[d2x ; d2y ; d2z];
%         d3P = [ d3x ; d3y ; d3z ];
%     case 7  % Les derivees sont a corriger
%         R=0.00*sin(f2*t) ; A=0.1270 ;
%         x=R*cos(f*t) ; y=R*sin(f*t) ;
%         z= A*sin(f2*t) -0.2 ;
%         dx=-f*R*sin(f*t) ; dy=f*R*cos(f*t)  ;  
%         dz= f2*A*cos(f2*t) ;
%         d2x=-f^2*R*cos(f*t) ; d2y=-f^2*R*sin(f*t)  ;
%         d2z = -f2^2*A*sin(f2*t) ;
%         P=[x ; y ; z];
%         dP=[dx ; dy ; dz];
%         d2P=[d2x ; d2y ; d2z];
%         % L'a _coup :
%         d3x=f^3*R*sin(f*t) ; d3y=-f^3*R*cos(f*t)  ;
%         d3z = -f2^3*A*cos(f2*t) ;
%         d3P=[d3x ; d3y ; d3z];
    case 8
        x=0 ; y=0 ; z=z0 ;
        P=[x ; y ; z];
        dP=[0 ; 0 ; 0];
        d2P=[0 ; 0 ; 0];
        d3P=[0 ; 0 ; 0];
        
    otherwise
        P=[0 ; 0 ; 0];
        dP=[0 ; 0 ; 0];
        d2P=[0 ; 0 ; 0];
        d3P = [ 0 ; 0 ; 0 ];
end
